simulink model "PID_Controller"  (R2020b)
settings: Solver=FixedStepAuto  StartTime=0.0  StopTime=0.2  FixedStep=0.004  RelTol=1e-3
values from neighbouring files (symbols this model uses):
  Ki = 500.0    [Problem4_data.sldd]
  Kp = 50.0    [Problem4_data.sldd]
  Ts = 0.0001    [Problem4_data.sldd]
settings Model: DataDictionary=Problem4_data.sldd  Creator=ASUS  LastModifiedBy=ASUS
settings SolverCC: AlgebraicLoopSolver=LineSearch
settings DataIOCC: SaveOutput=off  SaveTime=off

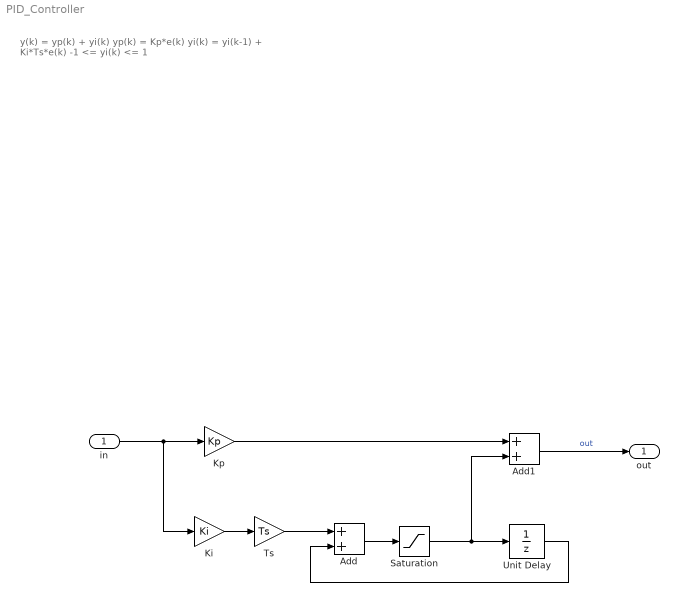
== system PID_Controller ==
  note: y(k) = yp(k) + yi(k)
      |
      | yp(k) = Kp*e(k)
      |
      | yi(k) = yi(k-1) + Ki*Ts*e(k)
      |
      | -1 <= yi(k) <= 1
  in : Inport  OutDataTypeStr=double  PortDimensions=1
  Add : Sum
  Add1 : Sum
  Ki : Gain  Gain=Ki
  Kp : Gain  Gain=Kp
  Saturation : Saturate  UpperLimit=1  LowerLimit=-1
  Ts : Gain  Gain=Ts
  Unit Delay : UnitDelay  SampleTime=-1  HasFrameUpgradeWarning=on
  out : Outport  OutDataTypeStr=double  PortDimensions=1  SampleTime=[0.0040000000000000001,0]
  wires:
  Kp/1 -> Add1/1
  Ki/1 -> Ts/1
  Add/1 -> Saturation/1
  in/1 -> Kp/1, Ki/1
  Ts/1 -> Add/1
  Unit Delay/1 -> Add/2
  Saturation/1 -> Unit Delay/1, Add1/2
  Add1/1 -> out/1  "out"
